simulink model "simulacionRobot"  (R2023b)
settings: Solver=ode45  StartTime=0.0  StopTime=30.0  RelTol=1e-3  EnableMultiTasking=on
values from neighbouring files (symbols this model uses):
  d = 1    [TrabajoTema6.m]    (also in simularRobot.m = 5)
  Lref = 0.5    [TrabajoTema6.m]    (also in simularRobot.m)
  phi_inicial = 0    [TrabajoTema6.m]    (also in simularRobot.m)
  R = 0.25    [TrabajoTema6.m]    (also in simularRobot.m)
  x = [x1,x2,x3]    [TrabajoTema6.m]    (also in simularRobot.m = 6 + radio * cos(theta))
  x_inicial = p0(1)    [TrabajoTema6.m]    (also in simularRobot.m = 2)
  y = [y1,y2,y3]    [TrabajoTema6.m]    (also in simularRobot.m = 7 + radio * sin(theta))
  y_inicial = p0(2)    [TrabajoTema6.m]    (also in simularRobot.m = 1)
settings Model: Creator=jalo  LastModifiedBy=alexo
settings SolverCC: AlgebraicLoopSolver=TrustRegion
settings DataIOCC: MaxDataPoints=100000  SaveFormat=Array  ReturnWorkspaceOutputs=off
settings OptimizationCC: LifeSpan=inf
settings DebuggingCC: UnconnectedInputMsg=warning  UnconnectedOutputMsg=warning  UnconnectedLineMsg=warning  SFUnexpectedBacktrackingDiag=warning  SFNoUnconditionalDefaultTransitionDiag=warning  SFExecutionAtInitializationDiag=none  ArithmeticOperatorsInVariantConditions=warning
settings HardwareCC: ProdBitPerPointer=32  ProdBitPerSizeT=32  ProdBitPerPtrDiffT=32  ProdLargestAtomicFloat=None  ProdIntDivRoundTo=Undefined  ProdEndianess=Unspecified  ProdWordSize=32  ProdHWDeviceType=32-bit Generic
settings ModelReferenceCC: EnableRefExpFcnMdlSchedulingChecks=on  PropagateSignalLabelsOutOfModel=off
settings SFSimCC: SimUseLocalCustomCode=off  CustomCodeUndefinedFunction=UseInterfaceOnly
settings RTWCC: RTWUseLocalCustomCode=off
settings CodeAppCC: StateflowObjectComments=on
settings GRTTargetCC: TargetLangStandard=C89/C90 (ANSI)
settings ConfigComp: CovMetricSettings=dw  CovSaveCumulativeToWorkspaceVar=on  CovSaveSingleToWorkspaceVar=on  CovExternalEMLEnable=off  CovSFcnEnable=off

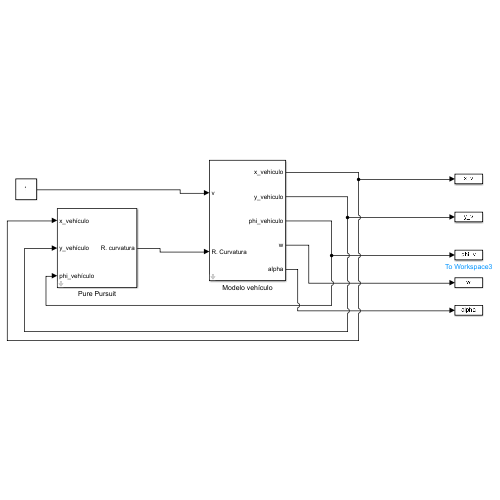
[thumbnail: Simulink's stored preview of the top-level diagram]
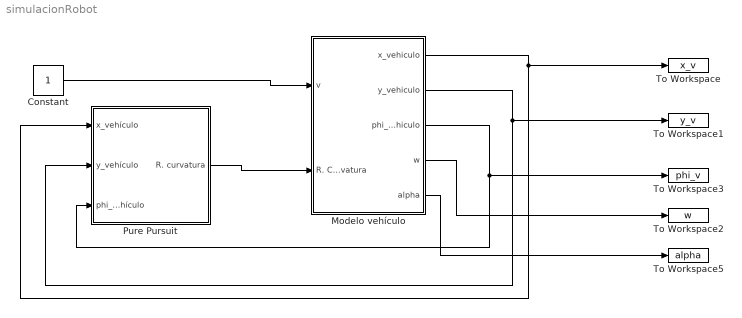
== system simulacionRobot ==
  Constant : Constant
  Modelo vehículo : Subsystem  mask{x0=x_inicial, y0=y_inicial, phi0=phi_inicial, d=d, R=R}
      mask prompts: x0 "Valor inicial de la coordenada x:"; y0 "Valor inicial de la coordenada y:"; phi0 "Valor inicial de la orientación:"; d "Distancia entre ejes"; R "Radio de la rueda"
  Pure Pursuit : Subsystem  mask(Pure Pursuit I){x_camino=x, y_camino=y, L=Lref}
      mask prompts: x_camino "Coordenadas x del camino:"; y_camino "Coordenadas y del camino:"; L "Parámetro Look-ahead (L):"
      mask help: Este bloque se encarga de calcular la curvatura que es necesario suministrar al vehículo cuando se emplea la técnica de persecución pura con el parámetro look-ahead (L) fijo.
      mask init:
      | global K_ANT
      | K_ANT=1;
  To Workspace : ToWorkspace  VariableName=x_v  SampleTime=-1
  To Workspace1 : ToWorkspace  VariableName=y_v  SampleTime=-1
  To Workspace2 : ToWorkspace  VariableName=w  SampleTime=-1
  To Workspace3 : ToWorkspace  VariableName=phi_v  SampleTime=-1
  To Workspace5 : ToWorkspace  VariableName=alpha  SampleTime=-1
  wires:
  Constant/1 -> Modelo vehículo/1(v)
  Pure Pursuit/1(R. curvatura) -> Modelo vehículo/2(R. Curvatura)
  Modelo vehículo/1(x_vehiculo) -> Pure Pursuit/1(x_vehículo), To Workspace/1
  Modelo vehículo/2(y_vehiculo) -> Pure Pursuit/2(y_vehículo), To Workspace1/1
  Modelo vehículo/3(phi_vehiculo) -> Pure Pursuit/3(phi_vehículo), To Workspace3/1
  Modelo vehículo/4(w) -> To Workspace2/1
  Modelo vehículo/5(alpha) -> To Workspace5/1

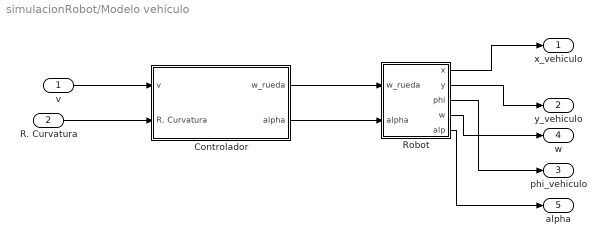
== system simulacionRobot/Modelo vehículo ==
  v : Inport
  R. Curvatura : Inport  Port=2
  Controlador : Subsystem
  Robot : Subsystem
  x_vehiculo : Outport
  y_vehiculo : Outport  Port=2
  phi_vehiculo : Outport  Port=3
  w : Outport  Port=4
  alpha : Outport  Port=5
  wires:
  Robot/1(x) -> x_vehiculo/1
  Robot/2(y) -> y_vehiculo/1
  Robot/3(phi) -> phi_vehiculo/1
  v/1 -> Controlador/1(v)
  R. Curvatura/1 -> Controlador/2(R. Curvatura)
  Controlador/1(w_rueda) -> Robot/1(w_rueda)
  Controlador/2(alpha) -> Robot/2(alpha)
  Robot/4(w) -> w/1
  Robot/5(alp) -> alpha/1

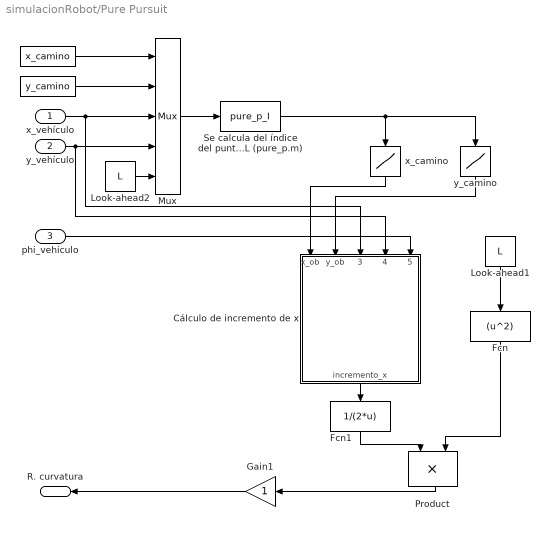
== system simulacionRobot/Pure Pursuit ==
  x_vehículo : Inport
  y_vehículo : Inport  Port=2
  phi_vehículo : Inport  Port=3
  " " : Constant  Value=y_camino
  "  " : Constant  Value=x_camino
  Cálculo de incremento de x : Subsystem
  Fcn : Fcn  Expr=(u^2)
  Fcn1 : Fcn  Expr=1/(2*u)
  Gain1 : Gain  SaturateOnIntegerOverflow=on  OutDataTypeStr=Inherit: Same as input  ParamDataTypeStr=Inherit: Same as input
  Look-ahead1 : Constant  Value=L
  Look-ahead2 : Constant  Value=L
  Mux : Mux  Inputs=5
  Product : Product  InputSameDT=on  RndMeth=Zero  SaturateOnIntegerOverflow=on  OutDataTypeStr=Inherit: Same as first input
  Se calcula del índice del punto que está a distancia L (pure_p.m) : MATLABFcn  MATLABFcn=pure_p_I
  x_camino : Lookup  InputValues=1:length(x_camino)  Table=x_camino
  y_camino : Lookup  InputValues=1:length(y_camino)  Table=y_camino
  R. curvatura : Outport
  wires:
  Fcn/1 -> Product/2
  Look-ahead1/1 -> Fcn/1
  Se calcula del índice del punto que está a distancia L (pure_p.m)/1 -> y_camino/1, x_camino/1
  y_camino/1 -> Cálculo de incremento de x/2(y_ob)
  x_camino/1 -> Cálculo de incremento de x/1(x_ob)
  Gain1/1 -> R. curvatura/1
  Product/1 -> Gain1/1
  "  "/1 -> Mux/1
  " "/1 -> Mux/2
  x_vehículo/1 -> Mux/3, Cálculo de incremento de x/3(x_vehículo)
  y_vehículo/1 -> Mux/4, Cálculo de incremento de x/4(y_vehículo)
  Look-ahead2/1 -> Mux/5
  Mux/1 -> Se calcula del índice del punto que está a distancia L (pure_p.m)/1
  phi_vehículo/1 -> Cálculo de incremento de x/5(phi_vehículo)
  Cálculo de incremento de x/1(incremento_x) -> Fcn1/1
  Fcn1/1 -> Product/1

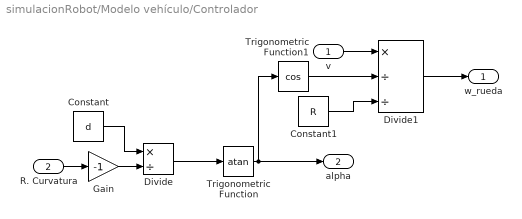
== system simulacionRobot/Modelo vehículo/Controlador ==
  v : Inport
  R. Curvatura : Inport  Port=2
  Constant : Constant  Value=d
  Constant1 : Constant  Value=R
  Divide : Product  Inputs=*/
  Divide1 : Product  Inputs=*//
  Gain : Gain  Gain=-1
  Trigonometric Function : Trigonometry  Operator=atan
  Trigonometric Function1 : Trigonometry  Operator=cos
  w_rueda : Outport
  alpha : Outport  Port=2
  wires:
  Constant/1 -> Divide/1
  Divide/1 -> Trigonometric Function/1
  Trigonometric Function/1 -> Trigonometric Function1/1, alpha/1
  v/1 -> Divide1/1
  Trigonometric Function1/1 -> Divide1/2
  Constant1/1 -> Divide1/3
  Divide1/1 -> w_rueda/1
  R. Curvatura/1 -> Gain/1
  Gain/1 -> Divide/2

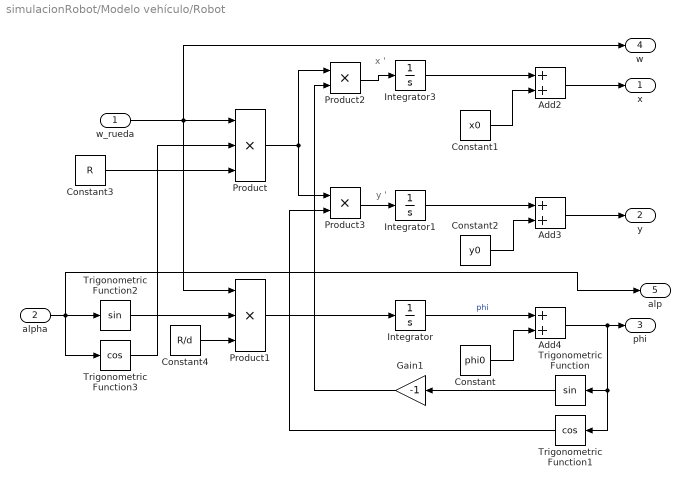
== system simulacionRobot/Modelo vehículo/Robot ==
  note: y '
  note: x '
  w_rueda : Inport
  alpha : Inport  Port=2
  Add2 : Sum
  Add3 : Sum
  Add4 : Sum
  Constant : Constant  Value=phi0
  Constant1 : Constant  Value=x0
  Constant2 : Constant  Value=y0
  Constant3 : Constant  Value=R
  Constant4 : Constant  Value=R/d
  Gain1 : Gain  Gain=-1
  Integrator : Integrator
  Integrator1 : Integrator
  Integrator3 : Integrator
  Product : Product  Inputs=3
  Product1 : Product  Inputs=3
  Product2 : Product
  Product3 : Product
  Trigonometric Function : Trigonometry
  Trigonometric Function1 : Trigonometry  Operator=cos
  Trigonometric Function2 : Trigonometry
  Trigonometric Function3 : Trigonometry  Operator=cos
  x : Outport
  y : Outport  Port=2
  phi : Outport  Port=3
  w : Outport  Port=4
  alp : Outport  Port=5
  wires:
  Integrator/1 -> Add4/1  "phi"
  Constant/1 -> Add4/2
  Add4/1 -> Trigonometric Function1/1, Trigonometric Function/1, phi/1
  Integrator3/1 -> Add2/1
  Constant1/1 -> Add2/2
  Add2/1 -> x/1
  Constant2/1 -> Add3/2
  Integrator1/1 -> Add3/1
  Add3/1 -> y/1
  alpha/1 -> Trigonometric Function3/1, Trigonometric Function2/1, alp/1
  w_rueda/1 -> w/1, Product1/1, Product/1
  Trigonometric Function3/1 -> Product/2
  Trigonometric Function2/1 -> Product1/2
  Constant3/1 -> Product/3
  Constant4/1 -> Product1/3
  Product1/1 -> Integrator/1
  Product/1 -> Product3/1, Product2/1
  Product3/1 -> Integrator1/1
  Product2/1 -> Integrator3/1
  Trigonometric Function1/1 -> Product3/2
  Trigonometric Function/1 -> Gain1/1
  Gain1/1 -> Product2/2

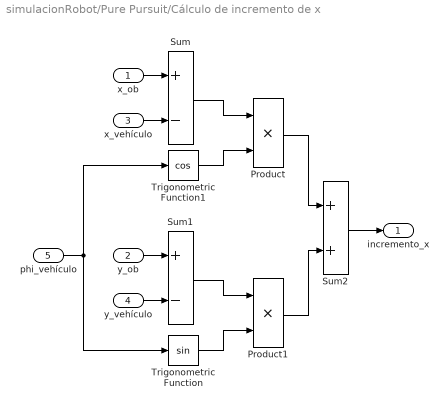
== system simulacionRobot/Pure Pursuit/Cálculo de incremento de x ==
  x_ob : Inport
  y_ob : Inport  Port=2
  x_vehículo : Inport  Port=3
  y_vehículo : Inport  Port=4
  phi_vehículo : Inport  Port=5
  Product : Product  InputSameDT=on  RndMeth=Zero  SaturateOnIntegerOverflow=on  OutDataTypeStr=Inherit: Same as first input
  Product1 : Product  InputSameDT=on  RndMeth=Zero  SaturateOnIntegerOverflow=on  OutDataTypeStr=Inherit: Same as first input
  Sum : Sum  Inputs=+-  InputSameDT=on  SaturateOnIntegerOverflow=on  OutDataTypeStr=Inherit: Same as first input
  Sum1 : Sum  Inputs=+-  InputSameDT=on  SaturateOnIntegerOverflow=on  OutDataTypeStr=Inherit: Same as first input
  Sum2 : Sum  InputSameDT=on  SaturateOnIntegerOverflow=on  OutDataTypeStr=Inherit: Same as first input
  Trigonometric Function : Trigonometry
  Trigonometric Function1 : Trigonometry  Operator=cos
  incremento_x : Outport
  wires:
  Sum2/1 -> incremento_x/1
  Product1/1 -> Sum2/2
  Product/1 -> Sum2/1
  Trigonometric Function/1 -> Product1/2
  Sum1/1 -> Product1/1
  phi_vehículo/1 -> Trigonometric Function/1, Trigonometric Function1/1
  Trigonometric Function1/1 -> Product/2
  Sum/1 -> Product/1
  y_vehículo/1 -> Sum1/2
  y_ob/1 -> Sum1/1
  x_vehículo/1 -> Sum/2
  x_ob/1 -> Sum/1
